simulink model "passivity_velmod_sim"  (R2020a)
settings: Solver=VariableStepAuto  StartTime=0.0  StopTime=T  FixedStep=dt  MaxStep=dtmax  RelTol=1e-3
values from neighbouring files (symbols this model uses):
  b = b*b_error_scale    (= 131.4)    [Hinf_run.m]    (also in adaptive_control_run.m; passivity_fmod_run.m; passivity_velmod_run.m)
  dt = 0.002    [adaptive_control_run.m]    (also in passivity_fmod_run.m; passivity_velmod_run.m)
  input_type = 3    [Hinf_run.m]    (also in adaptive_control_run.m; passivity_fmod_run.m; passivity_velmod_run.m)
  k = k*k_error_scale    (= 11691)    [Hinf_run.m]    (also in adaptive_control_run.m; passivity_fmod_run.m; passivity_velmod_run.m)
  m = 500    [Hinf_run.m]    (also in adaptive_control_run.m; passivity_fmod_run.m; passivity_velmod_run.m)
  rampslope = 0.1    [Hinf_run.m]    (also in adaptive_control_run.m; passivity_fmod_run.m; passivity_velmod_run.m)
  sineamp = 0.1    [Hinf_run.m]    (also in adaptive_control_run.m; passivity_fmod_run.m; passivity_velmod_run.m)
  sinefreq = pi/2    (= 1.57079632679)    [Hinf_run.m]    (also in adaptive_control_run.m; passivity_fmod_run.m; passivity_velmod_run.m)
  stepval = 0.1    [Hinf_run.m]    (also in adaptive_control_run.m; passivity_fmod_run.m; passivity_velmod_run.m)
  taum = taum*taum_error_scale    (= 0.108)    [Hinf_run.m]    (also in adaptive_control_run.m; passivity_fmod_run.m; passivity_velmod_run.m)
undefined symbols (not defined in the file or in its folder): DiscIntNeverNeededParam
settings Model: Creator=davidcarabis  LastModifiedBy=davidcarabis
settings DataIOCC: ReturnWorkspaceOutputs=off
settings DebuggingCC: ArithmeticOperatorsInVariantConditions=warning
settings SFSimCC: CustomCodeUndefinedFunction=UseInterfaceOnly

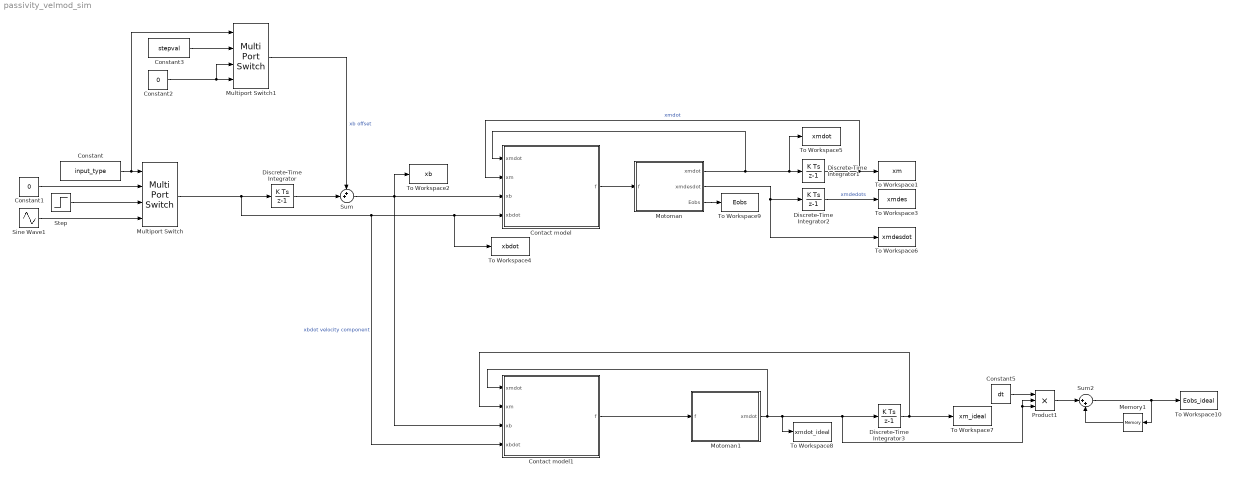
== system passivity_velmod_sim ==
  Constant : Constant  Value=input_type
  Constant1 : Constant  Value=0
  Constant2 : Constant  Value=0
  Constant3 : Constant  Value=stepval
  Constant5 : Constant  Value=dt
  Contact model : Subsystem
  Contact model1 : Subsystem
  Discrete-Time Integrator{,1..3} (4 alike) : DiscreteIntegrator  SampleTime=dt  ICPrevOutput=DiscIntNeverNeededParam  ICPrevScaledInput=DiscIntNeverNeededParam
  Memory1 : Memory
  Motoman : Subsystem
  Motoman1 : Subsystem
  Multiport Switch : MultiPortSwitch
  Multiport Switch1 : MultiPortSwitch
  Product1 : Product  Inputs=3
  Sine Wave1 : Sin  Amplitude=sineamp*sinefreq  Frequency=sinefreq  Phase=pi/2  SampleTime=0
  Step : Step  Time=0  After=rampslope  SampleTime=0
  Sum : Sum  Inputs=++|
  Sum2 : Sum  Inputs=|++
  To Workspace1 : ToWorkspace  VariableName=xm
  To Workspace10 : ToWorkspace  VariableName=Eobs_ideal
  To Workspace2 : ToWorkspace  VariableName=xb
  To Workspace3 : ToWorkspace  VariableName=xmdes
  To Workspace4 : ToWorkspace  VariableName=xbdot
  To Workspace5 : ToWorkspace  VariableName=xmdot
  To Workspace6 : ToWorkspace  VariableName=xmdesdot
  To Workspace7 : ToWorkspace  VariableName=xm_ideal
  To Workspace8 : ToWorkspace  VariableName=xmdot_ideal
  To Workspace9 : ToWorkspace  VariableName=Eobs
  wires:
  Multiport Switch/1 -> Discrete-Time Integrator/1, Contact model1/4(xbdot), To Workspace4/1, Contact model/4(xbdot)  "xbdot velocity component"
  Constant/1 -> Multiport Switch1/1, Multiport Switch/1
  Step/1 -> Multiport Switch/3
  Sine Wave1/1 -> Multiport Switch/4
  Constant1/1 -> Multiport Switch/2
  Multiport Switch1/1 -> Sum/1  "xb offset"
  Discrete-Time Integrator/1 -> Sum/2
  Constant2/1 -> Multiport Switch1/3, Multiport Switch1/4
  Constant3/1 -> Multiport Switch1/2
  Motoman/1(xmdot) -> To Workspace5/1, Discrete-Time Integrator1/1, Contact model/1(xmdot)
  Contact model/1(f) -> Motoman/1(f)
  Motoman/2(xmdesdot) -> Discrete-Time Integrator2/1, To Workspace6/1
  Motoman1/1(xmdot) -> To Workspace8/1, Product1/3, Product1/2, Discrete-Time Integrator3/1, Contact model1/1(xmdot)
  Contact model1/1(f) -> Motoman1/1(f)
  Discrete-Time Integrator3/1 -> Contact model1/2(xm), To Workspace7/1
  Discrete-Time Integrator2/1 -> To Workspace3/1  "xmdedots"
  Sum/1 -> Contact model/3(xb), To Workspace2/1, Contact model1/3(xb)
  Discrete-Time Integrator1/1 -> To Workspace1/1, Contact model/2(xm)  "xmdot"
  Product1/1 -> Sum2/1
  Sum2/1 -> Memory1/1, To Workspace10/1
  Constant5/1 -> Product1/1
  Memory1/1 -> Sum2/2
  Motoman/3(Eobs) -> To Workspace9/1

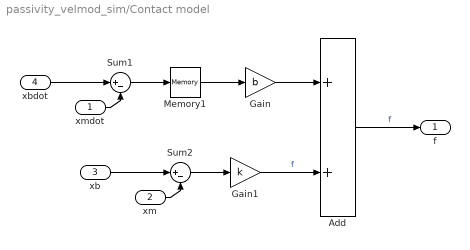
== system passivity_velmod_sim/Contact model ==
  xmdot : Inport
  xm : Inport  Port=2
  xb : Inport  Port=3
  xbdot : Inport  Port=4
  Add : Sum
  Gain : Gain  Gain=b
  Gain1 : Gain  Gain=k
  Memory1 : Memory
  Sum1 : Sum  Inputs=|+-
  Sum2 : Sum  Inputs=|+-
  f : Outport  VectorParamsAs1DForOutWhenUnconnected=off
  wires:
  Sum2/1 -> Gain1/1
  xb/1 -> Sum2/1
  xm/1 -> Sum2/2
  xmdot/1 -> Sum1/2
  xbdot/1 -> Sum1/1
  Gain/1 -> Add/1
  Sum1/1 -> Memory1/1
  Add/1 -> f/1  "f"
  Gain1/1 -> Add/2  "f"
  Memory1/1 -> Gain/1

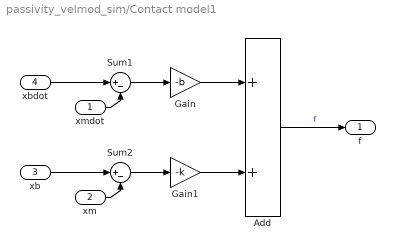
== system passivity_velmod_sim/Contact model1 ==
  xmdot : Inport
  xm : Inport  Port=2
  xb : Inport  Port=3
  xbdot : Inport  Port=4
  Add : Sum
  Gain : Gain  Gain=-b
  Gain1 : Gain  Gain=-k
  Sum1 : Sum  Inputs=|+-
  Sum2 : Sum  Inputs=|+-
  f : Outport  VectorParamsAs1DForOutWhenUnconnected=off
  wires:
  xmdot/1 -> Sum1/2
  Add/1 -> f/1  "f"
  Sum2/1 -> Gain1/1
  xb/1 -> Sum2/1
  Gain1/1 -> Add/2
  Sum1/1 -> Gain/1
  xbdot/1 -> Sum1/1
  Gain/1 -> Add/1
  xm/1 -> Sum2/2

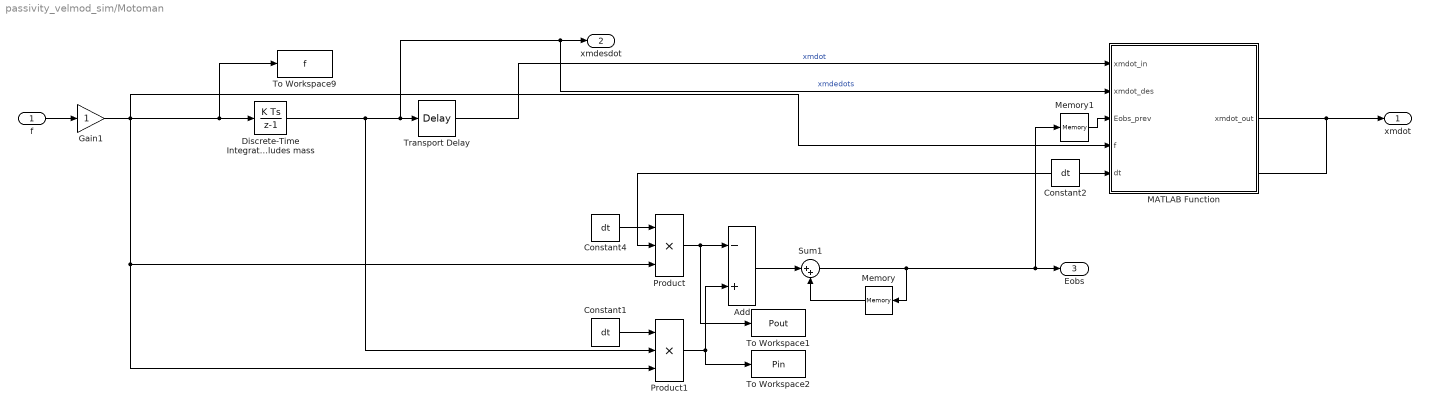
== system passivity_velmod_sim/Motoman ==
  f : Inport
  Add : Sum  Inputs=-+
  Constant1 : Constant  Value=dt
  Constant2 : Constant  Value=dt
  Constant4 : Constant  Value=dt
  Discrete-Time Integrator Includes mass : DiscreteIntegrator  gainval=1/m  SampleTime=dt  ICPrevOutput=DiscIntNeverNeededParam  ICPrevScaledInput=DiscIntNeverNeededParam
  Gain1 : Gain
  MATLAB Function : MATLAB Function  TreatAsAtomicUnit=on
  Memory : Memory
  Memory1 : Memory
  Product : Product  Inputs=3
  Product1 : Product  Inputs=3
  Sum1 : Sum  Inputs=|++
  To Workspace1 : ToWorkspace  VariableName=Pout
  To Workspace2 : ToWorkspace  VariableName=Pin
  To Workspace9 : ToWorkspace  VariableName=f
  Transport Delay : TransportDelay  DelayTime=taum
  xmdot : Outport  VectorParamsAs1DForOutWhenUnconnected=off
  xmdesdot : Outport  Port=2  VectorParamsAs1DForOutWhenUnconnected=off
  Eobs : Outport  Port=3  VectorParamsAs1DForOutWhenUnconnected=off
  wires:
  Discrete-Time Integrator Includes mass/1 -> Product1/2, MATLAB Function/2(xmdot_des), xmdesdot/1, Transport Delay/1  "xmdedots"
  Transport Delay/1 -> MATLAB Function/1(xmdot_in)  "xmdot"
  f/1 -> Gain1/1
  Memory/1 -> Sum1/2
  Constant4/1 -> Product/1
  Sum1/1 -> Memory1/1, Eobs/1, Memory/1
  Add/1 -> Sum1/1
  Product/1 -> To Workspace1/1, Add/1
  Constant1/1 -> Product1/1
  Product1/1 -> To Workspace2/1, Add/2
  MATLAB Function/1(xmdot_out) -> Product/2, xmdot/1
  Memory1/1 -> MATLAB Function/3(Eobs_prev)
  Constant2/1 -> MATLAB Function/5(dt)
  Gain1/1 -> MATLAB Function/4(f), To Workspace9/1, Discrete-Time Integrator Includes mass/1, Product1/3, Product/3

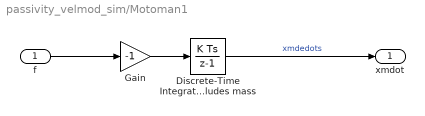
== system passivity_velmod_sim/Motoman1 ==
  f : Inport
  Discrete-Time Integrator Includes mass : DiscreteIntegrator  gainval=1/m  SampleTime=dt  ICPrevOutput=DiscIntNeverNeededParam  ICPrevScaledInput=DiscIntNeverNeededParam
  Gain : Gain  Gain=-1
  xmdot : Outport  VectorParamsAs1DForOutWhenUnconnected=off
  wires:
  Discrete-Time Integrator Includes mass/1 -> xmdot/1  "xmdedots"
  f/1 -> Gain/1
  Gain/1 -> Discrete-Time Integrator Includes mass/1

== matlab function passivity_velmod_sim/Motoman/MATLAB Function ==
  data: xmdot_in input; xmdot_out output; xmdot_des input; Eobs_prev input; f input; dt input
function xmdot_out = fcn(xmdot_in,xmdot_des,Eobs_prev,f,dt)

tol = 0.1;

Eobs = Eobs_prev + f*xmdot_des*dt - f*xmdot_in*dt;

% if (Eobs<0)&&(abs(f)>tol)
%     xmdot_out = (f*xmdot_des*dt - Eobs_prev)/(f*dt);
%     
% else
%     xmdot_out = xmdot_in;
% end


if (Eobs>0)&&(abs(f)>tol)
    xmdot_out = xmdot_in + Eobs_prev/(f*dt);
    %xmdot_out = xmdot_in;
else
    xmdot_out = xmdot_in;
end
